simulink model "VDP_Oscillator_syn"  (R2021a)
settings: Solver=VariableStepAuto  StartTime=0.0  StopTime=50  RelTol=1e-3
settings Model: Creator=JianFongLee  LastModifiedBy=JianFongLee

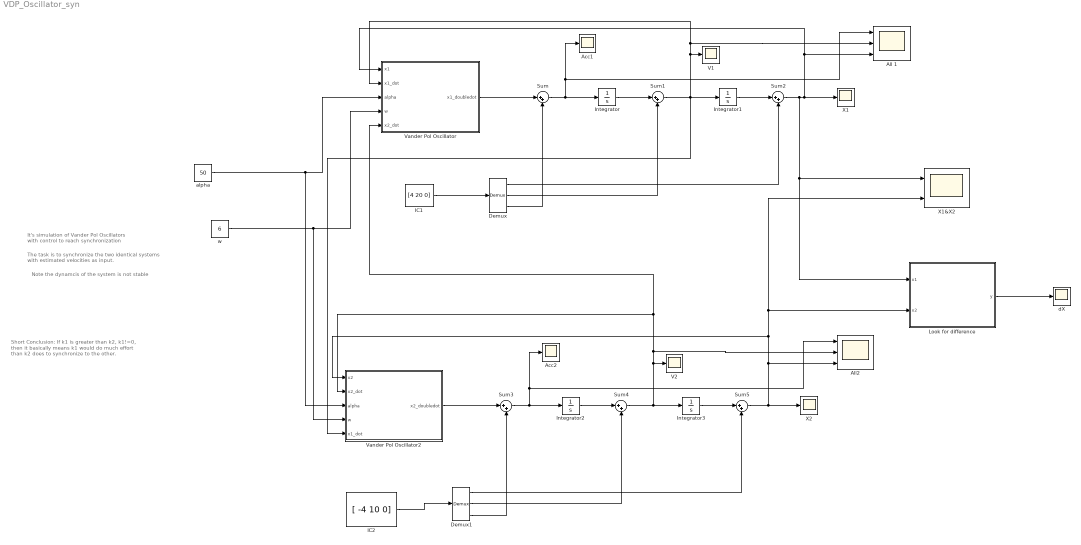
== system VDP_Oscillator_syn ==
  note: Short Conclusion:
      | If k1 is greater than k2, k1!=0,
      | then it basically means k1 would do much
      | effort than k2 does to synchronize to the other.
  note: Note the dynamcis of the system is not stable
  note: The task is to synchronize the two identical systems
      | with estimated velocities as input.
  note: It's simulation of Vander Pol Oscillators
      | with control to reach synchronization
  Acc1 : Scope
  Acc2 : Scope
  All 1 : Scope  NumInputPorts=3
  All2 : Scope  NumInputPorts=3
  Demux : Demux  Outputs=3
      settings: DisplayOption=none
  Demux1 : Demux  Outputs=3
      settings: DisplayOption=none
  IC1 : Constant  Value=[4 20 0]
  IC2 : Constant  Value=[ -4 10 0]
  Integrator{,1..3} (4 alike) : Integrator
  Look for difference : MATLAB Function  TreatAsAtomicUnit=on
  Sum{,1..5} (6 alike) : Sum  Inputs=|++
  V1 : Scope
  V2 : Scope
  Vander Pol Oscillator : MATLAB Function  TreatAsAtomicUnit=on
  Vander Pol Oscillator2 : MATLAB Function  TreatAsAtomicUnit=on
  X1 : Scope
  X1&X2 : Scope  NumInputPorts=2
  X2 : Scope
  alpha : Constant  Value=50
  dX : Scope
  w : Constant  Value=6
  wires:
  Integrator1/1 -> Sum2/1
  Sum/1 -> Acc1/1, All 1/1, Integrator/1
  Demux/1 -> Sum2/2
  Demux/2 -> Sum1/2
  Vander Pol Oscillator/1(x1_doubledot) -> Sum/1
  Integrator/1 -> Sum1/1
  Sum2/1 -> X1/1, Vander Pol Oscillator/1(x1), All 1/3, X1&X2/1, Look for difference/1(x1)
  IC1/1 -> Demux/1
  Demux/3 -> Sum/2
  Sum1/1 -> Vander Pol Oscillator2/5(x1_dot), V1/1, All 1/2, Vander Pol Oscillator/2(x1_dot), Integrator1/1
  Integrator3/1 -> Sum5/1
  alpha/1 -> Vander Pol Oscillator/3(alpha), Vander Pol Oscillator2/3(alpha)
  w/1 -> Vander Pol Oscillator/4(w), Vander Pol Oscillator2/4(w)
  Sum3/1 -> Acc2/1, All2/1, Integrator2/1
  Demux1/1 -> Sum5/2
  Demux1/2 -> Sum4/2
  Vander Pol Oscillator2/1(x2_doubledot) -> Sum3/1
  Integrator2/1 -> Sum4/1
  Sum5/1 -> X1&X2/2, Look for difference/2(x2), Vander Pol Oscillator2/1(x2), All2/3, X2/1
  IC2/1 -> Demux1/1
  Demux1/3 -> Sum3/2
  Sum4/1 -> Vander Pol Oscillator/5(x2_dot), Vander Pol Oscillator2/2(x2_dot), All2/2, V2/1, Integrator3/1
  Look for difference/1(y) -> dX/1

== matlab function VDP_Oscillator_syn/Vander Pol Oscillator ==
  data: x1 input; x1_doubledot output; x1_dot input; alpha input; w input; x2_dot input
function x1_doubledot = dynamics(x1,x1_dot,alpha,w,x2_dot)
%Parameters assignment
% alpha = 1;  %%% should be greater than 0
% w = 5;
k1 = 1.1; %%% k1+k2 should be greater than 1
x1_doubledot = -alpha*(x1^2-1)*x1_dot - w^2*x1 + alpha*k1*(x2_dot-x1_dot);
end

%%% Dynamics of Vander Pol Oscillator
%%% x1_doubledot + alpha*(x^2-1)*x1_dot + w^2*x1 = u;
%%% u = alpha*k1*(x2_dot - x1_dot)

== matlab function VDP_Oscillator_syn/Look for difference ==
  data: x1 input; y output; x2 input
function y = fcn(x1,x2)
%%% To see how mcuh they synch
y = x1 - x2;
end

== matlab function VDP_Oscillator_syn/Vander Pol Oscillator2 ==
  data: x2 input; x2_doubledot output; x2_dot input; alpha input; w input; x1_dot input
function x2_doubledot = dynamics(x2,x2_dot,alpha,w,x1_dot)
%Parameters assignment
% alpha = 1;  %%% should be greater than 0
% w = 5;
k2 = 1.2; %%% k1+k2 should be greater than 1
x2_doubledot = -alpha*(x2^2-1)*x2_dot - w^2*x2 + alpha*k2*(x1_dot-x2_dot);
%x2_doubledot = -alpha*(x2^2-1)*x2_dot - w^2*x2;

end

%%% Dynamics of Vander Pol Oscillator
%%% x2_doubledot + alpha*(x^2-1)*x2_dot + w^2*x2 = u;
%%% u = alpha*k2*(x1_dot - x2_dot)
